simulink model "Flight_Controllers"  (R2024a)
settings: Solver=VariableStepAuto  StartTime=0.0  StopTime=tFinal  FixedStep=0.02  RelTol=1e-3
values from neighbouring files (symbols this model uses):
  bOmega = -bThrust/mThrust    (= 168.963839792)    [Load_VehicleParams.m]
  Cant_cosine_Loss = cos(fanCantAngle)    [Load_VehicleParams.m]
  g = 9.807    [Load_VehicleParams.m]
  g_Offset = 5/6    (= 0.833333333333)    [Load_VehicleParams.m]
  Kd_LatPos = -0.04577    [Load_Controller_Gains_1.m]    (also in Load_Controller_Gains_13.m = -0.1; Load_Controller_Gains_2.m = 0.642; Load_Controller_Gains_3.m = -0.103; Load_Controller_Gains_4.m = 0)
  Kd_LatVel = 0    [Load_Controller_Gains_4.m]
  Kd_Pitch = 14.4    [Load_Controller_Gains_1.m]    (also in Load_Controller_Gains_13.m = 40; Load_Controller_Gains_2.m = 33; Load_Controller_Gains_3.m = 40; Load_Controller_Gains_4.m = 78.1)
  Ki_LatPos = -9.22e-6    (= -9.22e-06)    [Load_Controller_Gains_1.m]    (also in Load_Controller_Gains_13.m = 0.001; Load_Controller_Gains_2.m = 0.0199; Load_Controller_Gains_3.m = 0; Load_Controller_Gains_4.m = 0)
  Ki_LatVel = -0.00284    [Load_Controller_Gains_1.m]    (also in Load_Controller_Gains_2.m = -0.0122; Load_Controller_Gains_4.m = 0)
  Ki_Pitch = 3.17    [Load_Controller_Gains_4.m]
  Kp_LatPos = -0.0024    [Load_Controller_Gains_1.m]    (also in Load_Controller_Gains_13.m = -0.0248; Load_Controller_Gains_2.m = 1.53; Load_Controller_Gains_3.m = -0.0175; Load_Controller_Gains_4.m = 0.413)
  Kp_LatVel = -0.0296    [Load_Controller_Gains_1.m]    (also in Load_Controller_Gains_2.m = -0.059; Load_Controller_Gains_4.m = -0.291)
  Kp_Pitch = 5.36    [Load_Controller_Gains_1.m]    (also in Load_Controller_Gains_13.m = 38; Load_Controller_Gains_2.m = 24.8; Load_Controller_Gains_3.m = 38; Load_Controller_Gains_4.m = 43.7)
  mOmega = 1/mThrust    (= 1.62153397114)    [Load_VehicleParams.m]
  N_LatPos = 54.3    [Load_Controller_Gains_1.m]    (also in Load_Controller_Gains_13.m = 120; Load_Controller_Gains_2.m = 15.8; Load_Controller_Gains_3.m = 12; Load_Controller_Gains_4.m = 0)
  N_LatVel = 0    [Load_Controller_Gains_4.m]
  N_Pitch = 18.2    [Load_Controller_Gains_1.m]    (also in Load_Controller_Gains_13.m = 550; Load_Controller_Gains_2.m = 109; Load_Controller_Gains_3.m = 550; Load_Controller_Gains_4.m = 1115)
  nFans = 4    [Load_VehicleParams.m]
  pitch_Cmd_Limit = 7*pi/180    (= 0.12217304764)    [Load_Controller_Gains_13.m]    (also in Load_Controller_Gains_2.m = 0.10471975512; Load_Controller_Gains_3.m; Load_Controller_Gains_4.m)
  tau_LatPos = 0.2    [Load_Controller_Gains_1.m]    (also in Load_Controller_Gains_2.m = 0.01)
  tau_vCmd = 0.01    [Load_Controller_Gains_2.m]    (also in Load_Controller_Gains_4.m = 0.1)
  tau_xCmd = 0.2    [Load_Controller_Gains_3.m]
  Ts_Control = 1/50    (= 0.02)    [run_Lander_GNC_MonteCarloSim.m]
  vCmd_Integr_Limit = 0.25    [Load_Controller_Gains_2.m]
  velCmd_Limit = 2    [Load_Controller_Gains_2.m]    (also in Load_Controller_Gains_4.m = 0.12217304764)
undefined symbols (not defined in the file or in its folder): den_Gc_z_Pitch, den_Gc_z_Pos, num_Gc_z_Pitch, num_Gc_z_Pos, posCntrl_Integr_Limit
libraries: slpidlib x17
(part 3 of 3)

== matlab function Flight_Controllers/Vertical_Controller ==
  data: t input; fltSched input double; switchLines input; z_E input; zVel input; fireCmd output; Vertical_Mode output; Cntrl_telem output; m input; LandNowFl input
function [fireCmd, Vertical_Mode, Cntrl_telem] ... 
                                 = Control_Vert(t, fltSched, switchLines, z_E,zVel, m, LandNowFl)  
    %  Vertical Control Algotithm
    %    h is Altitude (m)
    %    hDot is Altitude Rate (m/s)
    %    hDot_Cmd is the Commanded Altitude Rate (m/s)
    %    m is the mass of the vehicle (kg)
    %    hyst_Width is the width of the hysteresis deadband (m/s)
    %          Will fire when vErr < -hyst_Width/2 and continue firing
    %          until vErr > hyst_Width/2.

validateattributes(t, {'double'}, {'scalar'})
validateattributes(LandNowFl, {'logical'}, {'scalar'})
% validateattributes(Xe, {'struct'}, {'scalar'})  % Bus becomes a Structure inside a Matlab function
% validateattributes(Vb, {'struct'}, {'scalar'})
% validateattributes(fltSched, {'numeric'}, {'column','numel',3})

% validateattributes(Xe, {'numeric'}, {'column','numel',3})  Used with Mux
%                                                       (NOT with a Bus)


velHyst = 0.20;  %   Hysteresis for the Vertical Velocity Phase Plane

persistent thr_previous
if isempty(thr_previous) 
    thr_previous = 0; % Initialize 
end

fireCmd = 0;

hErr = 0;   vErr = 0;


h = -1*z_E;  % m   "Z" position or the Altitude "h"
              %   Multiply by -1 because +Z is Down


hDot = -1*zVel;  % m/s   "Z" velocity or the Altitude rate "hDot"  (+Z is DOWN)



Vertical_Mode = interp1( fltSched(:,1), fltSched(:,2), t, 'previous');
vertCmd  = interp1( fltSched(:,1), fltSched(:,3), t, 'previous'); 

hCmd = 0;   hDot_Cmd = 0;

if Vertical_Mode == 1  % Mode 1 is Vertical Rate Control
    hDot_Cmd = vertCmd;
    hCmd = NaN;
    vErr = hDot - hDot_Cmd; % m/s  Velocity Error
    
    if vErr < -velHyst/2
        fireCmd = 1;
    elseif vErr > velHyst/2
        fireCmd = 0;
    else                           % You are in the Hysteresis Band
        if thr_previous > 0
            fireCmd = 1; % In the Hysteresis Band & Continue Firing
        else
            fireCmd = 0;  % Don't fire until you reach the bottom of the Hysteresis Band
        end
    end


elseif Vertical_Mode == 2   % Mode 2 is Vertical Postion Control (i.e. Hover)
    hCmd = vertCmd;
    hDot_Cmd = NaN;


   lowerSwitchLine = switchLines(  1: 4, :);  % See "run_AltitudePhasePlane_Design.m"
   lowerHystLine   = switchLines(  5:8, :);

   %% Find respective points on the upper & lower switch lines that correspond to hErr
   hErr = h - hCmd; % m/s  Altitude Error
   vErr = hDot - 0; % m/s  Velocity Error  (hDotCmd must = 0 for Postion Control)

   if hErr < lowerSwitchLine(1,1)  % In case h is outside the range of the PP design
       hErr = lowerSwitchLine(1,1);
   end
   if hErr > lowerSwitchLine(end,1)
       hErr = lowerSwitchLine(end,1);
end

%     formatSpec = '   t = %g  hErr = %g  vErr = %g';
%     str = sprintf(formatSpec, t, hErr, vErr)

hDot_err_lower = interpn( lowerSwitchLine(:,1), lowerSwitchLine(:,2), hErr );

hDot_err_lowerHyst = interpn( lowerHystLine(:,1), lowerHystLine(:,2), hErr );

%  Make Attitude Control Firing Decision   (Either Fire or don't and let gravity pull you down)
includeHysteresis = 1; %   Without hysteresis there is a risk you will rapidly pulse from
                       %      one side of a switch line to the other.
if includeHysteresis   %  ------------- With Hysteresis  -----------------
    
    if vErr < hDot_err_lower 
        fireCmd = 1;  % Fire the Center Cold Gas Engine
    
    elseif (vErr > hDot_err_lower) & (vErr < hDot_err_lowerHyst)
        fireCmd = thr_previous;  %   You are in the lower hysteresis band
   
    else fireCmd = 0;  % In the Drift zone
           fireCmd = 0;
    end

else  %    ----------------  No Hysteresis  -----------------------------
    if vErr < hDot_err_lower 
        fireCmd = 1;  % Fire
 
    else fireCmd = 0;  % In the Drift zone
    end
  end
end

% %  Display some data for debugging purposes.  Comment out when not needed.
% formatSpec = " Segment %2g  Prev Seg = %2g  t = %4g  t1 = %4g  t2 = %4g  VertVelCmd = %4g  VertPosCmd = %4g";
% str = sprintf(formatSpec, flightSegment, flightSegmentPrevious, t, t1, t2, VertVelCmd, VertPosCmd);
% disp(str)
%    formatSpec = "      LandNowFl = %2g ";
%    str = sprintf(formatSpec, single(LandNowFl) );
%    disp(str)


% Cntrl_telem = [t h hDot hDot_Cmd vErr thr_previous fireCmd];
Cntrl_telem = [t h hDot hDot_Cmd hCmd hErr vErr thr_previous fireCmd Vertical_Mode];

thr_previous = fireCmd;  % Set Previous Fire Command

== matlab function Flight_Controllers/Lateral_Controllers/Lateral_Control_3/Lateral_Flight_Plan ==
  data: xCmd output; t input; LatFlt_Schedule input
function xCmd  = Lateral_Schedule(t, LatFlt_Schedule)

%  For Controller version 3 there is only 1 Lateral Control Mode and that is
%    Position Control.  Velocity is "controlled" indirectly by how the
%    position command is structured.
%  The Lateral Flight Schedule is arranged as follows:
%        Column 1:  Time (sec)
%        Column 2:  Mode   Always Mode 2 for Position Control
%        Column 3:  xCmd   X Position Command
%        Column 4:  vLim   Currently NOT used

% validateattributes(t, {'double'}, {'scalar'})

xCmd  = interp1( LatFlt_Schedule(:,1), LatFlt_Schedule(:,3), t); 
% vLim  = interp1( LatFlt_Schedule(:,1), LatFlt_Schedule(:,4), t, 'previous'); 

% modeLat = 2; %  Always Postion Mode.  Keeping this so the plot script is 
             %     good for this and Control schemes with more than one
             %     mode.

== matlab function Flight_Controllers/Lateral_Controllers/Lateral_Control_4/Lateral_Flight_Plan ==
  data: xCmd output; t input; LatFlt_Schedule input

function xCmd  = Lateral_Schedule(t, LatFlt_Schedule)

%  For Controller version 4 there is only 1 Lateral Control Mode and that is
%    Position Control.  Velocity is "controlled" indirectly by how the
%    position command is structured.
%  The Lateral Flight Schedule is arranged as follows:
%        Column 1:  Time (sec)
%        Column 2:  Mode   Always Mode 2 for Position Control
%        Column 3:  xCmd   X Position Command
%        Column 4:  vLim   Currently NOT used

% validateattributes(t, {'double'}, {'scalar'})

xCmd  = interp1( LatFlt_Schedule(:,1), LatFlt_Schedule(:,3), t); 
% vLim  = interp1( LatFlt_Schedule(:,1), LatFlt_Schedule(:,4), t, 'previous'); 

% modeLat = 2; %  Always Postion Mode.  Keeping this so the plot script is 
             %     good for this and Control schemes with more than one
             %     mode.

== matlab function Flight_Controllers/Lateral_Controllers/Lateral_Control_13/Lateral_Flight_Plan ==
  data: xCmd output; t input; LatFlt_Schedule input
function xCmd  = Lateral_Schedule(t, LatFlt_Schedule)

%  For Controller version 3 there is only 1 Lateral Control Mode and that is
%    Position Control.  Velocity is "controlled" indirectly by how the
%    position command is structured.
%  The Lateral Flight Schedule is arranged as follows:
%        Column 1:  Time (sec)
%        Column 2:  Mode   Always Mode 2 for Position Control
%        Column 3:  xCmd   X Position Command
%        Column 4:  vLim   Currently NOT used

% validateattributes(t, {'double'}, {'scalar'})

xCmd  = interp1( LatFlt_Schedule(:,1), LatFlt_Schedule(:,3), t); 
% vLim  = interp1( LatFlt_Schedule(:,1), LatFlt_Schedule(:,4), t, 'previous'); 

% modeLat = 2; %  Always Postion Mode.  Keeping this so the plot script is 
             %     good for this and Control schemes with more than one
             %     mode.

== matlab function Flight_Controllers/Lateral_Controllers/Lateral_Control_2/Lateral_Flight_Plan ==
  data: modeLat output; xCmd output; t input; vLim output; LatFlt_Schedule input
function [modeLat, xCmd, vLim] = Lateral_Schedule(t, LatFlt_Schedule)

%  For Controller version 2 there is only 1 Lateral Control Mode and that is
%    Position Control.  Velocity is "controlled" by a LIMIT on the
%    veloctity command coming from the Position Controller
%  The Lateral Flight Schedule is arranged as follows:
%        Column 1:  Time (sec)
%        Column 2:  Mode   Mode 1 is Velocity Control,  Mode 2 is Position Control
%        Column 3:  xCmd   X velocity command if in mode 1,  Position if in mode 2
%        Column 4:  vLim   X Velocity Limit

% validateattributes(t, {'double'}, {'scalar'})

xCmd  = interp1( LatFlt_Schedule(:,1), LatFlt_Schedule(:,3), t, 'previous'); 
vLim  = interp1( LatFlt_Schedule(:,1), LatFlt_Schedule(:,4), t, 'previous'); 

modeLat = 2; %  Always Postion Mode.  Keeping this so the plot script is 
             %     good for this and Control schemes with more than one
             %     mode.

== matlab function Flight_Controllers/Lateral_Controllers/Lateral_Control_1/Lateral_Flight_Plan ==
  data: t input; modeLat output; LatFlt_Schedule input; xCmd output; yCmd output
function [modeLat, xCmd, yCmd] = Lateral_Schedule(t, LatFlt_Schedule)

%  There are 2 Lateral Control Modes:  Velocity and Position
%  The Lateral Flight Schedule is arranged as follows:
%        Column 1:  Time (sec)
%        Column 2:  Mode   Mode 1 is Velocity Control,  Mode 2 is Position Control
%        Column 3:  xCmd   X velocity command if in mode 1,  Position if in mode 2
%        Column 4:  yCmd   Y velocity command if in mode 1,  Position if in mode 2

% validateattributes(t, {'double'}, {'scalar'})


modeLat = interp1( LatFlt_Schedule(:,1), LatFlt_Schedule(:,2), t, 'previous');
xCmd  = interp1( LatFlt_Schedule(:,1), LatFlt_Schedule(:,3), t, 'previous'); 
yCmd  = interp1( LatFlt_Schedule(:,1), LatFlt_Schedule(:,4), t, 'previous');

== matlab function Flight_Controllers/Lateral_Controllers/Lateral_Control_1/MATLAB Function ==
  data: Lat_Mode input; Vel_on_off output; Pos_on_off output
function [Vel_on_off, Pos_on_off] = fcn(Lat_Mode)

%   Mode 1 is Lateral Velocity Control,  Mode 2 is Lateral Position Control

if Lat_Mode > 1.5   %  Turn Position ON and Velocity OFF
    Vel_on_off = -1;  % Negative so Enabled System for velocity doesn't run
    Pos_on_off = 1;
else                   %  Turn Velocity ON and Positio OFF
    Vel_on_off =  1;  
    Pos_on_off = -1;  % Negative so Enabled System for position doesn't run
end

== matlab function Flight_Controllers/Lateral_Controllers/Lateral_Control_14/Lateral_Flight_Plan ==
  data: xCmd output; t input; LatFlt_Schedule input

function xCmd  = Lateral_Schedule(t, LatFlt_Schedule)

%  For Controller version 4 there is only 1 Lateral Control Mode and that is
%    Position Control.  Velocity is "controlled" indirectly by how the
%    position command is structured.
%  The Lateral Flight Schedule is arranged as follows:
%        Column 1:  Time (sec)
%        Column 2:  Mode   Always Mode 2 for Position Control
%        Column 3:  xCmd   X Position Command
%        Column 4:  vLim   Currently NOT used

% validateattributes(t, {'double'}, {'scalar'})

xCmd  = interp1( LatFlt_Schedule(:,1), LatFlt_Schedule(:,3), t); 
% vLim  = interp1( LatFlt_Schedule(:,1), LatFlt_Schedule(:,4), t, 'previous'); 

% modeLat = 2; %  Always Postion Mode.  Keeping this so the plot script is 
             %     good for this and Control schemes with more than one
             %     mode.
